simulink model "Grid_SensorLayout_SpatialAllignment_Clustering"  (R2018a)
settings: Solver=FixedStepAuto  StartTime=0.0  StopTime=SimulationTime  FixedStep=SamplingTime  RelTol=1e-3
values from neighbouring files (symbols this model uses):
  ValidateGRID = true    [SensorFusion_Script0_main.m]
  ValidateLAYOUT = true    [SensorFusion_Script0_main.m]
  VisualizeCLUSTERING = true    [SensorFusion_Script0_main.m]
undefined symbols (not defined in the file or in its folder): ACTIVATE_CAM, ACTIVATE_RAD, CAM1_detTimeStamp, CAM1_MeasNoise, CAM1_objClassID, CAM1_PX, CAM1_PY, CAM1_VX, CAM1_VY, CAM2_detTimeStamp, CAM2_MeasNoise, CAM2_objClassID, CAM2_PX, CAM2_PY, CAM2_VX, CAM2_VY, CAM3_detTimeStamp, CAM3_MeasNoise, CAM3_objClassID, CAM3_PX, CAM3_PY, CAM3_VX, CAM3_VY, CAM4_detTimeStamp, CAM4_MeasNoise, CAM4_objClassID, CAM4_PX, CAM4_PY, CAM4_VX, CAM4_VY, CAM5_detTimeStamp, CAM5_MeasNoise, CAM5_objClassID, CAM5_PX, CAM5_PY, CAM5_VX, CAM5_VY, CAM6_detTimeStamp, CAM6_MeasNoise, CAM6_objClassID, CAM6_PX, CAM6_PY, CAM6_VX, CAM6_VY, CAM7_detTimeStamp, CAM7_MeasNoise, CAM7_objClassID, CAM7_PX, CAM7_PY, CAM7_VX, CAM7_VY, CAM8_detTimeStamp, CAM8_MeasNoise, CAM8_objClassID, CAM8_PX, CAM8_PY, CAM8_VX, CAM8_VY, CAM_nMeas, CAM_TYPE ... (+171)
libraries: simulink_extras x4
(part 3 of 10)

== system Grid_SensorLayout_SpatialAllignment_Clustering/SENSOR_MEASUREMENTS/RADAR_CAMERA_EGO_SENSOR_INTERFACE/RoadSensors/LineSensor2 ==
  timeIdx : Inport
  nLines : Inport  Port=2
  CameraLineCoeff : Inport  Port=3
  ExtractMeasParam1 : Subsystem
  For Iterator : ForIterator  ResetStates=reset  IterationSource=external  IterationVariableDataType=int16
  IsValid2 : Subsystem
  Selector : Selector  InputPortWidth=nCameras  IndexOptions=Index vector (dialog)  Indices=2  OutputSizes=1
  Subsystem1 : Subsystem
  C1 : Outport
  wires:
  ExtractMeasParam1/7(xmax) -> Subsystem1/9(xmax)
  ExtractMeasParam1/8(lineMarkWidth) -> Subsystem1/10(lineWidth)
  [index] -> IsValid2/1(LineID), Subsystem1/12(iter), ExtractMeasParam1/1(idx)
  timeIdx/1 -> ExtractMeasParam1/2(time)
  ExtractMeasParam1/2(curvRate) -> IsValid2/3(curvatureRate), [curvRate]
  [curvRate] -> Subsystem1/3(curvRate)
  [curv] -> Subsystem1/2(curv)
  ExtractMeasParam1/3(curvLength) -> IsValid2/4(curvLength), [curvLen]
  ExtractMeasParam1/1(curvature) -> IsValid2/2(curvature), [curv]
  Subsystem1/1(C1) -> C1/1
  [curvLen] -> Subsystem1/4(curvLen)
  For Iterator/1 -> [index]
  ExtractMeasParam1/4(headingAngle) -> IsValid2/5(HeadingAngle), [alpha]
  ExtractMeasParam1/5(lateralOffset) -> Subsystem1/7(lateralOffset)
  Selector/1 -> For Iterator/1
  IsValid2/1(validID) -> Subsystem1/6(ValidID)
  ExtractMeasParam1/6(xmin) -> Subsystem1/8(xmin)
  CameraLineCoeff/1 -> Subsystem1/1(CameraLineCoeff)
  nLines/1 -> Selector/1
  ExtractMeasParam1/9(measCaptureTime) -> Subsystem1/11(TIME_STAMP)
  [alpha] -> Subsystem1/5(alpha)

== system Grid_SensorLayout_SpatialAllignment_Clustering/SENSOR_MEASUREMENTS/RADAR_CAMERA_EGO_SENSOR_INTERFACE/RoadSensors/LineSensor3 ==
  timeIdx : Inport
  nLines : Inport  Port=2
  CameraLineCoeff : Inport  Port=3
  ExtractMeasParam1 : Subsystem
  For Iterator : ForIterator  ResetStates=reset  IterationSource=external  IterationVariableDataType=int16
  IsValid2 : Subsystem
  Selector : Selector  InputPortWidth=nCameras  IndexOptions=Index vector (dialog)  Indices=3  OutputSizes=1
  Subsystem1 : Subsystem
  C1 : Outport
  wires:
  ExtractMeasParam1/7(xmax) -> Subsystem1/9(xmax)
  ExtractMeasParam1/8(lineMarkWidth) -> Subsystem1/10(lineWidth)
  [index] -> IsValid2/1(LineID), Subsystem1/12(iter), ExtractMeasParam1/1(idx)
  timeIdx/1 -> ExtractMeasParam1/2(time)
  ExtractMeasParam1/2(curvRate) -> IsValid2/3(curvatureRate), [curvRate]
  [curvRate] -> Subsystem1/3(curvRate)
  [curv] -> Subsystem1/2(curv)
  ExtractMeasParam1/3(curvLength) -> IsValid2/4(curvLength), [curvLen]
  ExtractMeasParam1/1(curvature) -> IsValid2/2(curvature), [curv]
  Subsystem1/1(C1) -> C1/1
  [curvLen] -> Subsystem1/4(curvLen)
  For Iterator/1 -> [index]
  ExtractMeasParam1/4(headingAngle) -> IsValid2/5(HeadingAngle), [alpha]
  ExtractMeasParam1/5(lateralOffset) -> Subsystem1/7(lateralOffset)
  Selector/1 -> For Iterator/1
  IsValid2/1(validID) -> Subsystem1/6(ValidID)
  ExtractMeasParam1/6(xmin) -> Subsystem1/8(xmin)
  CameraLineCoeff/1 -> Subsystem1/1(CameraLineCoeff)
  nLines/1 -> Selector/1
  ExtractMeasParam1/9(measCaptureTime) -> Subsystem1/11(TIME_STAMP)
  [alpha] -> Subsystem1/5(alpha)

== system Grid_SensorLayout_SpatialAllignment_Clustering/SENSOR_MEASUREMENTS/RADAR_CAMERA_EGO_SENSOR_INTERFACE/RoadSensors/LineSensor4 ==
  timeIdx : Inport
  nLines : Inport  Port=2
  CameraLineCoeff : Inport  Port=3
  ExtractMeasParam1 : Subsystem
  For Iterator : ForIterator  ResetStates=reset  IterationSource=external  IterationVariableDataType=int16
  IsValid2 : Subsystem
  Selector : Selector  InputPortWidth=nCameras  IndexOptions=Index vector (dialog)  Indices=4  OutputSizes=1
  Subsystem1 : Subsystem
  C1 : Outport
  wires:
  ExtractMeasParam1/7(xmax) -> Subsystem1/9(xmax)
  ExtractMeasParam1/8(lineMarkWidth) -> Subsystem1/10(lineWidth)
  [index] -> IsValid2/1(LineID), Subsystem1/12(iter), ExtractMeasParam1/1(idx)
  timeIdx/1 -> ExtractMeasParam1/2(time)
  ExtractMeasParam1/2(curvRate) -> IsValid2/3(curvatureRate), [curvRate]
  [curvRate] -> Subsystem1/3(curvRate)
  [curv] -> Subsystem1/2(curv)
  ExtractMeasParam1/3(curvLength) -> IsValid2/4(curvLength), [curvLen]
  ExtractMeasParam1/1(curvature) -> IsValid2/2(curvature), [curv]
  Subsystem1/1(C1) -> C1/1
  [curvLen] -> Subsystem1/4(curvLen)
  For Iterator/1 -> [index]
  ExtractMeasParam1/4(headingAngle) -> IsValid2/5(HeadingAngle), [alpha]
  ExtractMeasParam1/5(lateralOffset) -> Subsystem1/7(lateralOffset)
  Selector/1 -> For Iterator/1
  IsValid2/1(validID) -> Subsystem1/6(ValidID)
  ExtractMeasParam1/6(xmin) -> Subsystem1/8(xmin)
  CameraLineCoeff/1 -> Subsystem1/1(CameraLineCoeff)
  nLines/1 -> Selector/1
  ExtractMeasParam1/9(measCaptureTime) -> Subsystem1/11(TIME_STAMP)
  [alpha] -> Subsystem1/5(alpha)

== system Grid_SensorLayout_SpatialAllignment_Clustering/SENSOR_MEASUREMENTS/RADAR_CAMERA_EGO_SENSOR_INTERFACE/RoadSensors/LineSensor5 ==
  timeIdx : Inport
  nLines : Inport  Port=2
  CameraLineCoeff : Inport  Port=3
  ExtractMeasParam1 : Subsystem
  For Iterator : ForIterator  ResetStates=reset  IterationSource=external  IterationVariableDataType=int16
  IsValid2 : Subsystem
  Selector : Selector  InputPortWidth=nCameras  IndexOptions=Index vector (dialog)  Indices=5  OutputSizes=1
  Subsystem1 : Subsystem
  C1 : Outport
  wires:
  ExtractMeasParam1/7(xmax) -> Subsystem1/9(xmax)
  ExtractMeasParam1/8(lineMarkWidth) -> Subsystem1/10(lineWidth)
  [index] -> IsValid2/1(LineID), Subsystem1/12(iter), ExtractMeasParam1/1(idx)
  timeIdx/1 -> ExtractMeasParam1/2(time)
  ExtractMeasParam1/2(curvRate) -> IsValid2/3(curvatureRate), [curvRate]
  [curvRate] -> Subsystem1/3(curvRate)
  [curv] -> Subsystem1/2(curv)
  ExtractMeasParam1/3(curvLength) -> IsValid2/4(curvLength), [curvLen]
  ExtractMeasParam1/1(curvature) -> IsValid2/2(curvature), [curv]
  Subsystem1/1(C1) -> C1/1
  [curvLen] -> Subsystem1/4(curvLen)
  For Iterator/1 -> [index]
  ExtractMeasParam1/4(headingAngle) -> IsValid2/5(HeadingAngle), [alpha]
  ExtractMeasParam1/5(lateralOffset) -> Subsystem1/7(lateralOffset)
  Selector/1 -> For Iterator/1
  IsValid2/1(validID) -> Subsystem1/6(ValidID)
  ExtractMeasParam1/6(xmin) -> Subsystem1/8(xmin)
  CameraLineCoeff/1 -> Subsystem1/1(CameraLineCoeff)
  nLines/1 -> Selector/1
  ExtractMeasParam1/9(measCaptureTime) -> Subsystem1/11(TIME_STAMP)
  [alpha] -> Subsystem1/5(alpha)

== system Grid_SensorLayout_SpatialAllignment_Clustering/SENSOR_MEASUREMENTS/RADAR_CAMERA_EGO_SENSOR_INTERFACE/RoadSensors/LineSensor6 ==
  timeIdx : Inport
  nLines : Inport  Port=2
  CameraLineCoeff : Inport  Port=3
  ExtractMeasParam1 : Subsystem
  For Iterator : ForIterator  ResetStates=reset  IterationSource=external  IterationVariableDataType=int16
  IsValid2 : Subsystem
  Selector : Selector  InputPortWidth=nCameras  IndexOptions=Index vector (dialog)  Indices=6  OutputSizes=1
  Subsystem1 : Subsystem
  C1 : Outport
  wires:
  ExtractMeasParam1/7(xmax) -> Subsystem1/9(xmax)
  ExtractMeasParam1/8(lineMarkWidth) -> Subsystem1/10(lineWidth)
  [index] -> IsValid2/1(LineID), Subsystem1/12(iter), ExtractMeasParam1/1(idx)
  timeIdx/1 -> ExtractMeasParam1/2(time)
  ExtractMeasParam1/2(curvRate) -> IsValid2/3(curvatureRate), [curvRate]
  [curvRate] -> Subsystem1/3(curvRate)
  [curv] -> Subsystem1/2(curv)
  ExtractMeasParam1/3(curvLength) -> IsValid2/4(curvLength), [curvLen]
  ExtractMeasParam1/1(curvature) -> IsValid2/2(curvature), [curv]
  Subsystem1/1(C1) -> C1/1
  [curvLen] -> Subsystem1/4(curvLen)
  For Iterator/1 -> [index]
  ExtractMeasParam1/4(headingAngle) -> IsValid2/5(HeadingAngle), [alpha]
  ExtractMeasParam1/5(lateralOffset) -> Subsystem1/7(lateralOffset)
  Selector/1 -> For Iterator/1
  IsValid2/1(validID) -> Subsystem1/6(ValidID)
  ExtractMeasParam1/6(xmin) -> Subsystem1/8(xmin)
  CameraLineCoeff/1 -> Subsystem1/1(CameraLineCoeff)
  nLines/1 -> Selector/1
  ExtractMeasParam1/9(measCaptureTime) -> Subsystem1/11(TIME_STAMP)
  [alpha] -> Subsystem1/5(alpha)

== system Grid_SensorLayout_SpatialAllignment_Clustering/SENSOR_MEASUREMENTS/RADAR_CAMERA_EGO_SENSOR_INTERFACE/RoadSensors/LineSensor7 ==
  timeIdx : Inport
  nLines : Inport  Port=2
  CameraLineCoeff : Inport  Port=3
  ExtractMeasParam1 : Subsystem
  For Iterator : ForIterator  ResetStates=reset  IterationSource=external  IterationVariableDataType=int16
  IsValid2 : Subsystem
  Selector : Selector  InputPortWidth=nCameras  IndexOptions=Index vector (dialog)  Indices=7  OutputSizes=1
  Subsystem1 : Subsystem
  C1 : Outport
  wires:
  ExtractMeasParam1/7(xmax) -> Subsystem1/9(xmax)
  ExtractMeasParam1/8(lineMarkWidth) -> Subsystem1/10(lineWidth)
  [index] -> IsValid2/1(LineID), Subsystem1/12(iter), ExtractMeasParam1/1(idx)
  timeIdx/1 -> ExtractMeasParam1/2(time)
  ExtractMeasParam1/2(curvRate) -> IsValid2/3(curvatureRate), [curvRate]
  [curvRate] -> Subsystem1/3(curvRate)
  [curv] -> Subsystem1/2(curv)
  ExtractMeasParam1/3(curvLength) -> IsValid2/4(curvLength), [curvLen]
  ExtractMeasParam1/1(curvature) -> IsValid2/2(curvature), [curv]
  Subsystem1/1(C1) -> C1/1
  [curvLen] -> Subsystem1/4(curvLen)
  For Iterator/1 -> [index]
  ExtractMeasParam1/4(headingAngle) -> IsValid2/5(HeadingAngle), [alpha]
  ExtractMeasParam1/5(lateralOffset) -> Subsystem1/7(lateralOffset)
  Selector/1 -> For Iterator/1
  IsValid2/1(validID) -> Subsystem1/6(ValidID)
  ExtractMeasParam1/6(xmin) -> Subsystem1/8(xmin)
  CameraLineCoeff/1 -> Subsystem1/1(CameraLineCoeff)
  nLines/1 -> Selector/1
  ExtractMeasParam1/9(measCaptureTime) -> Subsystem1/11(TIME_STAMP)
  [alpha] -> Subsystem1/5(alpha)

== system Grid_SensorLayout_SpatialAllignment_Clustering/SENSOR_MEASUREMENTS/RADAR_CAMERA_EGO_SENSOR_INTERFACE/RoadSensors/LineSensor8 ==
  timeIdx : Inport
  nLines : Inport  Port=2
  CameraLineCoeff : Inport  Port=3
  ExtractMeasParam1 : Subsystem
  For Iterator : ForIterator  ResetStates=reset  IterationSource=external  IterationVariableDataType=int16
  IsValid2 : Subsystem
  Selector : Selector  InputPortWidth=nCameras  IndexOptions=Index vector (dialog)  Indices=8  OutputSizes=1
  Subsystem1 : Subsystem
  C1 : Outport
  wires:
  ExtractMeasParam1/7(xmax) -> Subsystem1/9(xmax)
  ExtractMeasParam1/8(lineMarkWidth) -> Subsystem1/10(lineWidth)
  [index] -> IsValid2/1(LineID), Subsystem1/12(iter), ExtractMeasParam1/1(idx)
  timeIdx/1 -> ExtractMeasParam1/2(time)
  ExtractMeasParam1/2(curvRate) -> IsValid2/3(curvatureRate), [curvRate]
  [curvRate] -> Subsystem1/3(curvRate)
  [curv] -> Subsystem1/2(curv)
  ExtractMeasParam1/3(curvLength) -> IsValid2/4(curvLength), [curvLen]
  ExtractMeasParam1/1(curvature) -> IsValid2/2(curvature), [curv]
  Subsystem1/1(C1) -> C1/1
  [curvLen] -> Subsystem1/4(curvLen)
  For Iterator/1 -> [index]
  ExtractMeasParam1/4(headingAngle) -> IsValid2/5(HeadingAngle), [alpha]
  ExtractMeasParam1/5(lateralOffset) -> Subsystem1/7(lateralOffset)
  Selector/1 -> For Iterator/1
  IsValid2/1(validID) -> Subsystem1/6(ValidID)
  ExtractMeasParam1/6(xmin) -> Subsystem1/8(xmin)
  CameraLineCoeff/1 -> Subsystem1/1(CameraLineCoeff)
  nLines/1 -> Selector/1
  ExtractMeasParam1/9(measCaptureTime) -> Subsystem1/11(TIME_STAMP)
  [alpha] -> Subsystem1/5(alpha)

== system Grid_SensorLayout_SpatialAllignment_Clustering/OBJECT_TRACKER_SENSOR_FUSION/NEAREST_NEIGHBOUR_FOR_CAMERA_MEASUREMENT_GROUPING/NN_MEASUREMENT_GROUPING_WITHIN_EPS/COMPUTE_MEAN_IF_CLUSTER_FORMED/COMPUTE_COVARIANCE1 ==
  covariance_sum : Inport
  n : Inport  Port=2
  Constant : Constant  Value=uint16(1)
  Constant1 : Constant  Value=uint16(0)
  Constant2 : Constant  Value=single(eye(2))
  Constant3 : Constant  Value=single(0.001)
  Divide : Product  Inputs=*/
  LessThanOrEqual : RelationalOperator  Operator=>  OutDataTypeStr=boolean  RndMeth=Simplest
  LessThanOrEqual1 : RelationalOperator  Operator=<=  OutDataTypeStr=boolean  RndMeth=Simplest
  Logical Operator : Logic  AllPortsSameDT=off  OutDataTypeStr=boolean
  Selector : Selector  NumberOfDimensions=2  InputPortWidth=3  IndexOptions=Index vector (dialog),Index vector (dialog)  Indices=1,1  OutputSizes=1,1
  Selector1 : Selector  NumberOfDimensions=2  InputPortWidth=3  IndexOptions=Index vector (dialog),Index vector (dialog)  Indices=1,1  OutputSizes=1,1
  Subtract : Sum  Inputs=-+
  Switch : Switch  Criteria=u2 > Threshold  Threshold=uint16(1)
  Switch1 : Switch  Criteria=u2 > Threshold  Threshold=uint16(1)
  Covariance : Outport
  wires:
  n/1 -> [nPts], Switch/2
  Constant/1 -> Switch/1
  covariance_sum/1 -> Divide/1
  Constant1/1 -> Switch/3
  Switch/1 -> Subtract/1
  [nPts] -> Subtract/2
  Subtract/1 -> Divide/2
  Logical Operator/1 -> Switch1/2
  Switch1/1 -> Covariance/1
  Constant2/1 -> Switch1/3
  Divide/1 -> Selector1/1, Switch1/1, Selector/1
  Selector/1 -> LessThanOrEqual/1
  Selector1/1 -> LessThanOrEqual1/2
  Constant3/1 -> LessThanOrEqual1/1, LessThanOrEqual/2
  LessThanOrEqual/1 -> Logical Operator/1
  LessThanOrEqual1/1 -> Logical Operator/2

== system Grid_SensorLayout_SpatialAllignment_Clustering/OBJECT_TRACKER_SENSOR_FUSION/NEAREST_NEIGHBOUR_FOR_CAMERA_MEASUREMENT_GROUPING/NN_MEASUREMENT_GROUPING_WITHIN_EPS/COMPUTE_MEAN_IF_CLUSTER_FORMED/COMPUTE_COVARIANCE_SUM ==
  mean : Inport
  MeasArray : Inport  Port=2
  nPoints : Inport  Port=3
  ClusterMembers : Inport  Port=4
  Add1 : Sum
  Bus Selector : BusSelector  OutputSignals=MeasArray
  For Iterator : ForIterator  ResetStates=reset  IterationSource=external
  Matrix Multiply : Product  Multiplication=Matrix(*)
  Selector : Selector  NumberOfDimensions=2  InputPortWidth=3  IndexOptions=Select all,Index vector (port)  Indices=[1 3],1  OutputSizes=1,1
  Selector1 : Selector  NumberOfDimensions=2  InputPortWidth=3  IndexOptions=Select all,Index vector (port)  Indices=[1 3],1  OutputSizes=1,1
  Subtract : Sum  Inputs=+-
  Transpose : Math  Operator=transpose  SaturateOnIntegerOverflow=on
  Unit Delay : UnitDelay  InitialCondition=single(zeros(2,2))  SampleTime=-1
  ClusterCovSUM : Outport
  wires:
  nPoints/1 -> For Iterator/1
  ClusterMembers/1 -> Selector/1
  For Iterator/1 -> Selector/2
  MeasArray/1 -> Bus Selector/1
  Bus Selector/1 -> Selector1/1  "<MeasArray>"
  Selector/1 -> Selector1/2
  Unit Delay/1 -> Add1/1
  Add1/1 -> Unit Delay/1, ClusterCovSUM/1
  Subtract/1 -> Matrix Multiply/1, Transpose/1
  Transpose/1 -> Matrix Multiply/2
  Matrix Multiply/1 -> Add1/2
  Selector1/1 -> Subtract/2
  mean/1 -> Subtract/1

== system Grid_SensorLayout_SpatialAllignment_Clustering/OBJECT_TRACKER_SENSOR_FUSION/NEAREST_NEIGHBOUR_FOR_CAMERA_MEASUREMENT_GROUPING/NN_MEASUREMENT_GROUPING_WITHIN_EPS/COMPUTE_MEAN_IF_CLUSTER_FORMED/COMPUTE_MEAN ==
  mean_sum : Inport
  n : Inport  Port=2
  Divide : Product  Inputs=*/
  mean : Outport
  wires:
  mean_sum/1 -> Divide/1
  Divide/1 -> mean/1
  n/1 -> Divide/2

== system Grid_SensorLayout_SpatialAllignment_Clustering/OBJECT_TRACKER_SENSOR_FUSION/NEAREST_NEIGHBOUR_FOR_CAMERA_MEASUREMENT_GROUPING/NN_MEASUREMENT_GROUPING_WITHIN_EPS/COMPUTE_MEAN_IF_CLUSTER_FORMED/COMPUTE_MEAN_SUM ==
  ClusterMembers : Inport
  nPoints : Inport  Port=2
  MeasArray : Inport  Port=3
  Add1 : Sum
  Bus Selector : BusSelector  OutputSignals=MeasArray
  For Iterator : ForIterator  ResetStates=reset  IterationSource=external
  Selector : Selector  NumberOfDimensions=2  InputPortWidth=3  IndexOptions=Select all,Index vector (port)  Indices=[1 3],1  OutputSizes=1,1
  Selector1 : Selector  NumberOfDimensions=2  InputPortWidth=3  IndexOptions=Select all,Index vector (port)  Indices=[1 3],1  OutputSizes=1,1
  Unit Delay : UnitDelay  InitialCondition=single(0)  SampleTime=-1
  ClusterMeanSUM : Outport
  wires:
  nPoints/1 -> For Iterator/1
  ClusterMembers/1 -> Selector/1
  For Iterator/1 -> Selector/2
  MeasArray/1 -> Bus Selector/1
  Bus Selector/1 -> Selector1/1  "<MeasArray>"
  Selector/1 -> Selector1/2
  Selector1/1 -> Add1/2
  Unit Delay/1 -> Add1/1
  Add1/1 -> ClusterMeanSUM/1, Unit Delay/1

== system Grid_SensorLayout_SpatialAllignment_Clustering/OBJECT_TRACKER_SENSOR_FUSION/NEAREST_NEIGHBOUR_FOR_CAMERA_MEASUREMENT_GROUPING/NN_MEASUREMENT_GROUPING_WITHIN_EPS/COMPUTE_MEAN_IF_CLUSTER_FORMED/GET_DATA ==
  CLSTR : Inport
  Bus Selector : BusSelector  OutputSignals=ClusterSizes,nClusters,ClusterMember
  Selector : Selector  NumberOfDimensions=2  InputPortWidth=3  IndexOptions=Select all,Index vector (port)  Indices=[1 3],1  OutputSizes=1,1
  nPts : Outport
  <ClusterMember> : Outport  Port=2
  wires:
  Bus Selector/1 -> Selector/1  "<ClusterSizes>"
  Selector/1 -> nPts/1
  Bus Selector/2 -> Selector/2  "<nClusters>"
  Bus Selector/3 -> <ClusterMember>/1  "<ClusterMember>"
  CLSTR/1 -> Bus Selector/1

== system Grid_SensorLayout_SpatialAllignment_Clustering/OBJECT_TRACKER_SENSOR_FUSION/NEAREST_NEIGHBOUR_FOR_CAMERA_MEASUREMENT_GROUPING/NN_MEASUREMENT_GROUPING_WITHIN_EPS/For Iterator Subsystem/If Action Subsystem ==
  CLSTR_DATA : Inport
  Action Port : ActionPort  ActionType=else
  Constant : Constant  Value=uint16(0)
  CLSTR_DATA_NO_UPD : Outport
  nPtsEpsNoUpd : Outport  Port=2
  wires:
  CLSTR_DATA/1 -> CLSTR_DATA_NO_UPD/1
  Constant/1 -> nPtsEpsNoUpd/1

== system Grid_SensorLayout_SpatialAllignment_Clustering/OBJECT_TRACKER_SENSOR_FUSION/NEAREST_NEIGHBOUR_FOR_CAMERA_MEASUREMENT_GROUPING/NN_MEASUREMENT_GROUPING_WITHIN_EPS/For Iterator Subsystem/MERGE_SIGNALS ==
  CLSTR_NO_UPD : Inport
  nPtsEpsNoUpd : Inport  Port=2
  nPtsUpd : Inport  Port=3
  CLSTR_UPD : Inport  Port=4
  Merge : Merge
  Merge1 : Merge
  nPtsEps : Outport
  CLSTR_DATA : Outport  Port=2
  wires:
  CLSTR_NO_UPD/1 -> Merge1/1
  Merge1/1 -> CLSTR_DATA/1
  nPtsEpsNoUpd/1 -> Merge/1
  Merge/1 -> nPtsEps/1
  nPtsUpd/1 -> Merge/2
  CLSTR_UPD/1 -> Merge1/2

== system Grid_SensorLayout_SpatialAllignment_Clustering/OBJECT_TRACKER_SENSOR_FUSION/NEAREST_NEIGHBOUR_FOR_CAMERA_MEASUREMENT_GROUPING/NN_MEASUREMENT_GROUPING_WITHIN_EPS/For Iterator Subsystem/NN ==
  CLSTR_DATA : Inport  OutDataTypeStr=Bus: CLUSTER_DATA_STRUCT_SNSR
  measArray : Inport  Port=2
  idx_i : Inport  Port=3
  Action Port : ActionPort  ActionType=then
  PERFORM_NN_CLUSTERING : Subsystem
  SET_CLUSTER_ID_AND_UPDATE_NUMBER_OF_CLUSTERS : Subsystem
  Subsystem : Subsystem
  nPtsEps : Outport
  CLSTR_DATA_UPD : Outport  Port=2
  wires:
  idx_i/1 -> PERFORM_NN_CLUSTERING/4(idx_i)
  SET_CLUSTER_ID_AND_UPDATE_NUMBER_OF_CLUSTERS/2(CLUSTER_DATA) -> PERFORM_NN_CLUSTERING/3(CLSTR_DATA)
  SET_CLUSTER_ID_AND_UPDATE_NUMBER_OF_CLUSTERS/1(nRadMeas) -> PERFORM_NN_CLUSTERING/1(nMeas)
  CLSTR_DATA/1 -> SET_CLUSTER_ID_AND_UPDATE_NUMBER_OF_CLUSTERS/1(CLUSTERING_DATA)
  measArray/1 -> SET_CLUSTER_ID_AND_UPDATE_NUMBER_OF_CLUSTERS/2(CAM_MEAS_CTS), [meas]
  [meas] -> PERFORM_NN_CLUSTERING/2(measArray)
  Subsystem/1(ClstrSize) -> nPtsEps/1
  PERFORM_NN_CLUSTERING/1(CLSTR_DATA_UPD) -> Subsystem/1(CLSTR_DATA), CLSTR_DATA_UPD/1

== system Grid_SensorLayout_SpatialAllignment_Clustering/OBJECT_TRACKER_SENSOR_FUSION/NEAREST_NEIGHBOUR_FOR_CAMERA_MEASUREMENT_GROUPING/NN_MEASUREMENT_GROUPING_WITHIN_EPS/For Iterator Subsystem/Subsystem ==
  idx_i : Inport
  CLSTR_in : Inport  Port=2
  Bus Selector : BusSelector  OutputSignals=isMeasVisitedFlag
  Logical Operator1 : Logic  Operator=NOT  AllPortsSameDT=off  OutDataTypeStr=boolean
  Selector1 : Selector  NumberOfDimensions=2  InputPortWidth=3  IndexOptions=Select all,Index vector (port)  Indices=1,1  OutputSizes=1,1
  Unit Delay : UnitDelay  InitialCondition=CLSTR_SNSR_DELAY_INIT  SampleTime=-1
  isNotVisited : Outport
  CLSTR_out : Outport  Port=2
  wires:
  Logical Operator1/1 -> isNotVisited/1
  Selector1/1 -> Logical Operator1/1
  idx_i/1 -> Selector1/2
  CLSTR_in/1 -> Unit Delay/1
  Bus Selector/1 -> Selector1/1  "<isMeasVisitedFlag>"
  Unit Delay/1 -> CLSTR_out/1, Bus Selector/1

== system Grid_SensorLayout_SpatialAllignment_Clustering/OBJECT_TRACKER_SENSOR_FUSION/NEAREST_NEIGHBOUR_FOR_CAMERA_MEASUREMENT_GROUPING/NN_MEASUREMENT_GROUPING_WITHIN_EPS/Subsystem3/GET_DATA_FROM_BUS ==
  CLSTR_DATA : Inport
  Bus Selector : BusSelector  OutputSignals=ClusterCenter,ClusterCovariance,nClusters
  <ClusterCenter> : Outport
  <ClusterCovariance> : Outport  Port=2
  <nClusters> : Outport  Port=3
  wires:
  Bus Selector/3 -> <nClusters>/1  "<nClusters>"
  Bus Selector/1 -> <ClusterCenter>/1  "<ClusterCenter>"
  CLSTR_DATA/1 -> Bus Selector/1
  Bus Selector/2 -> <ClusterCovariance>/1  "<ClusterCovariance>"

== system Grid_SensorLayout_SpatialAllignment_Clustering/OBJECT_TRACKER_SENSOR_FUSION/NEAREST_NEIGHBOUR_FOR_CAMERA_MEASUREMENT_GROUPING/NN_MEASUREMENT_GROUPING_WITHIN_EPS/Subsystem3/SET_DATA_TO_BUS ==
  CLSTR_DATA : Inport
  Mean_ARRAY : Inport  Port=2
  Cov_ARRAY : Inport  Port=3
  Bus Creator : BusCreator  Inputs=7  OutDataTypeStr=Bus: CLUSTER_DATA_STRUCT_SNSR  NonVirtualBus=on
      settings: InheritFromInputs=off
  Bus Selector1 : BusSelector  OutputSignals=ClusterCenter,ClusterCovariance,ClusterSizes,ClusterToMeasAssignment,isMeasVisitedFlag,nClusters,ClusterMember
  Constant1 : Constant  Value=ClusterMemArray_SNSR
  Reshape1 : Reshape  OutputDimensionality=Row vector (2-D)
  Terminator1 : Terminator
  Terminator2 : Terminator
  Terminator3 : Terminator
  "CLSTR_DATA_UPD " : Outport
  wires:
  Constant1/1 -> Reshape1/1  "ClusterMember"
  Bus Selector1/5 -> Bus Creator/5  "<isMeasVisitedFlag>"
  Cov_ARRAY/1 -> Bus Creator/2  "ClusterCovariance"
  Mean_ARRAY/1 -> Bus Creator/1  "ClusterCenter"
  Bus Selector1/1 -> Terminator2/1  "<ClusterCenter>"
  Bus Selector1/7 -> Terminator1/1  "<ClusterMember>"
  Bus Selector1/2 -> Terminator3/1  "<ClusterCovariance>"
  Bus Selector1/3 -> Bus Creator/3  "<ClusterSizes>"
  Reshape1/1 -> Bus Creator/7  "ClusterMember"
  Bus Selector1/4 -> Bus Creator/4  "<ClusterToMeasAssignment>"
  Bus Selector1/6 -> Bus Creator/6  "<nClusters>"
  Bus Creator/1 -> "CLSTR_DATA_UPD "/1
  CLSTR_DATA/1 -> Bus Selector1/1

== system Grid_SensorLayout_SpatialAllignment_Clustering/OBJECT_TRACKER_SENSOR_FUSION/NEAREST_NEIGHBOUR_FOR_CAMERA_MEASUREMENT_GROUPING/NN_MEASUREMENT_GROUPING_WITHIN_EPS/Subsystem3/UPDATE_CLUSTER_DATA ==
  Center_ARRAY : Inport
  Cov_ARRAY : Inport  Port=2
  ID : Inport  Port=3
  mean1 : Inport  Port=4
  mean2 : Inport  Port=5
  Cov1 : Inport  Port=6
  Cov2 : Inport  Port=7
  FLAG : Inport  Port=8
  Assignment : Assignment  NumberOfDimensions=2  DiagnosticForDimensions=Warning  IndexOptions=Assign all,Index vector (port)  Indices=1,1  OutputSizes=1,1
  Assignment1 : Assignment  NumberOfDimensions=3  DiagnosticForDimensions=Warning  IndexOptions=Assign all,Assign all,Index vector (port)  Indices=1,1,1  OutputSizes=1,1,1
  Merge : Merge
  Merge2 : Merge
  Selector : Selector  NumberOfDimensions=2  InputPortWidth=3  IndexOptions=Select all,Index vector (port)  Indices=[1 3],1  OutputSizes=1,1
  Selector1 : Selector  NumberOfDimensions=3  InputPortWidth=3  IndexOptions=Select all,Select all,Index vector (port)  Indices=[1 3],1,1  OutputSizes=1,1,1
  Switch : Switch  Criteria=u2 ~= 0
  Switch1 : Switch  Criteria=u2 ~= 0
  CenterUpd : Outport
  CovUpd : Outport  Port=2
  wires:
  Selector/1 -> Switch/3
  Merge2/1 -> Switch1/1
  Cov_ARRAY/1 -> Assignment1/1, Selector1/1
  mean1/1 -> Merge/1
  Selector1/1 -> Switch1/3
  Merge/1 -> Switch/1
  Switch1/1 -> Assignment1/2
  Switch/1 -> Assignment/2
  Cov2/1 -> Merge2/2
  Assignment1/1 -> CovUpd/1
  Assignment/1 -> CenterUpd/1
  Cov1/1 -> Merge2/1
  mean2/1 -> Merge/2
  FLAG/1 -> [FLAG]
  [FLAG] -> Switch/2
  [FLAG] -> Switch1/2
  [ID] -> Assignment/3, Selector/2
  ID/1 -> [ID], Assignment1/3, Selector1/2
  Center_ARRAY/1 -> Selector/1, Assignment/1

== system Grid_SensorLayout_SpatialAllignment_Clustering/OBJECT_TRACKER_SENSOR_FUSION/SENSOR_LAYOUT_AND_CHRACTERIZATION/PRE_COMPUTE_SENSOR_FOV_GRID/COMPUTE_CAMERA_SNSR_GRID/ComputeCoverageANDConfidence ==
  RegionConfidenceArray : Inport
  nGridCells : Inport  Port=2
  GridIDVector : Inport  Port=3
  GridParam : Inport  Port=4
  SensorID : Inport  Port=5
  SensorExtrinsic : Inport  Port=6
  SensorIntrinsic : Inport  Port=7
  FOVOverlapArray : Inport  Port=8
  Compute_Cell_X_and_Y_index : Subsystem
  For Iterator : ForIterator  ResetStates=reset  IterationSource=external
  SET_DATA : Subsystem
  RegionConfidence : Outport
  FOVOverlap : Outport  Port=2
  wires:
  nGridCells/1 -> For Iterator/1
  For Iterator/1 -> SET_DATA/1(GridIndex), Compute_Cell_X_and_Y_index/1(CellIndex)
  GridParam/1 -> Compute_Cell_X_and_Y_index/3(GridParam)
  GridIDVector/1 -> Compute_Cell_X_and_Y_index/2(GridID_vec)
  SensorExtrinsic/1 -> Compute_Cell_X_and_Y_index/4(SensorExtrinsicParam)
  SensorIntrinsic/1 -> Compute_Cell_X_and_Y_index/5(SensorIntrinsicParam)
  RegionConfidenceArray/1 -> SET_DATA/2(RegionConfiArray)
  Compute_Cell_X_and_Y_index/1(RegionConfidence) -> SET_DATA/5(confi)
  SensorID/1 -> SET_DATA/4(SnsrIndex)
  FOVOverlapArray/1 -> SET_DATA/3(FOVOverlapArray)
  Compute_Cell_X_and_Y_index/2(FOVOverlap) -> SET_DATA/6(overlap)
  SET_DATA/1(RegionConfidence) -> RegionConfidence/1
  SET_DATA/2(FOVOverlap) -> FOVOverlap/1

== system Grid_SensorLayout_SpatialAllignment_Clustering/OBJECT_TRACKER_SENSOR_FUSION/SENSOR_LAYOUT_AND_CHRACTERIZATION/PRE_COMPUTE_SENSOR_FOV_GRID/COMPUTE_CAMERA_SNSR_GRID/GET_SENSOR_PARAMETERS ==
  SensorID : Inport
  SensorParam : Inport  Port=2
  Bus Selector : BusSelector  OutputSignals=CameraIntrinsics,CameraExtrinsics
  Bus Selector1 : BusSelector  OutputSignals=CameraType
  Selector : Selector  NumberOfDimensions=2  InputPortWidth=3  IndexOptions=Select all,Index vector (port)  Indices=[1 3],1  OutputSizes=1,1
  Selector1 : Selector  NumberOfDimensions=2  InputPortWidth=3  IndexOptions=Select all,Index vector (port)  Indices=[1 3],1  OutputSizes=1,1
  extrinsic : Outport
  intrinsic : Outport  Port=2
  wires:
  Bus Selector/2 -> Selector/1  "<CameraExtrinsics>"
  Bus Selector1/1 -> Selector1/2  "<CameraType>"
  Selector/1 -> extrinsic/1, Bus Selector1/1
  SensorID/1 -> Selector/2
  SensorParam/1 -> Bus Selector/1
  Bus Selector/1 -> Selector1/1  "<CameraIntrinsics>"
  Selector1/1 -> intrinsic/1

== system Grid_SensorLayout_SpatialAllignment_Clustering/OBJECT_TRACKER_SENSOR_FUSION/SENSOR_LAYOUT_AND_CHRACTERIZATION/PRE_COMPUTE_SENSOR_FOV_GRID/COMPUTE_RADAR_SNSR_GRID/ComputeCoverageANDConfidence ==
  RegionConfidenceArray : Inport
  nGridCells : Inport  Port=2
  GridIDVector : Inport  Port=3
  GridParam : Inport  Port=4
  SensorID : Inport  Port=5
  SensorExtrinsic : Inport  Port=6
  SensorIntrinsic : Inport  Port=7
  FOVOverlapArray : Inport  Port=8
  Compute_Cell_X_and_Y_index : Subsystem
  For Iterator : ForIterator  ResetStates=reset  IterationSource=external
  SET_DATA : Subsystem
  RegionConfidence : Outport
  FOVOverlap : Outport  Port=2
  wires:
  nGridCells/1 -> For Iterator/1
  For Iterator/1 -> SET_DATA/1(GridIndex), Compute_Cell_X_and_Y_index/1(CellIndex)
  GridParam/1 -> Compute_Cell_X_and_Y_index/3(GridParam)
  GridIDVector/1 -> Compute_Cell_X_and_Y_index/2(GridID_vec)
  SensorExtrinsic/1 -> Compute_Cell_X_and_Y_index/4(SensorExtrinsicParam)
  SensorIntrinsic/1 -> Compute_Cell_X_and_Y_index/5(SensorIntrinsicParam)
  RegionConfidenceArray/1 -> SET_DATA/2(RegionConfiArray)
  Compute_Cell_X_and_Y_index/1(RegionConfidence) -> SET_DATA/5(confi)
  SensorID/1 -> SET_DATA/4(SnsrIndex)
  FOVOverlapArray/1 -> SET_DATA/3(FOVOverlapArray)
  Compute_Cell_X_and_Y_index/2(FOVOverlap) -> SET_DATA/6(overlap)
  SET_DATA/1(RegionConfidence) -> RegionConfidence/1
  SET_DATA/2(FOVOverlap) -> FOVOverlap/1

== system Grid_SensorLayout_SpatialAllignment_Clustering/OBJECT_TRACKER_SENSOR_FUSION/SENSOR_LAYOUT_AND_CHRACTERIZATION/PRE_COMPUTE_SENSOR_FOV_GRID/COMPUTE_RADAR_SNSR_GRID/GET_SENSOR_PARAMETERS ==
  SensorID : Inport
  SensorParam : Inport  Port=2
  Bus Selector : BusSelector  OutputSignals=RadarIntrinsics,RadarExtrinsics
  Bus Selector1 : BusSelector  OutputSignals=RadarType
  Selector : Selector  NumberOfDimensions=2  InputPortWidth=3  IndexOptions=Select all,Index vector (port)  Indices=[1 3],1  OutputSizes=1,1
  Selector1 : Selector  NumberOfDimensions=2  InputPortWidth=3  IndexOptions=Select all,Index vector (port)  Indices=[1 3],1  OutputSizes=1,1
  extrinsic : Outport
  intrinsic : Outport  Port=2
  wires:
  Bus Selector/2 -> Selector/1  "<RadarExtrinsics>"
  Bus Selector1/1 -> Selector1/2  "<RadarType>"
  Selector/1 -> extrinsic/1, Bus Selector1/1
  SensorID/1 -> Selector/2
  SensorParam/1 -> Bus Selector/1
  Bus Selector/1 -> Selector1/1  "<RadarIntrinsics>"
  Selector1/1 -> intrinsic/1

== system Grid_SensorLayout_SpatialAllignment_Clustering/OBJECT_TRACKER_SENSOR_FUSION/SENSOR_LAYOUT_AND_CHRACTERIZATION/PRE_COMPUTE_SENSOR_FOV_GRID/CREATE_GRID/For Iterator Subsystem ==
  xIndex : Inport
  Cy : Inport  Port=2
  GridParam : Inport  Port=3
  CellIDArray : Inport  Port=4
  Compute_Grid_Cell_Cartesian_Coordinate : Subsystem
  Compute_Grid_Cell_Discreete_Index : Subsystem
  For Iterator : ForIterator  ResetStates=reset  IterationSource=external
  SET_DATA : Subsystem
  Terminator : Terminator
  Terminator1 : Terminator
  CellIDVectorUpd : Outport
  wires:
  Cy/1 -> For Iterator/1
  xIndex/1 -> Compute_Grid_Cell_Cartesian_Coordinate/2(x_Index)
  GridParam/1 -> Compute_Grid_Cell_Cartesian_Coordinate/1(GridParam), Compute_Grid_Cell_Discreete_Index/1(GridParam)
  Compute_Grid_Cell_Cartesian_Coordinate/2(y_Coordinate) -> Compute_Grid_Cell_Discreete_Index/3(y_coord)
  Compute_Grid_Cell_Cartesian_Coordinate/1(x_Coordinate) -> Compute_Grid_Cell_Discreete_Index/2(x_coord)
  For Iterator/1 -> Compute_Grid_Cell_Cartesian_Coordinate/3(y_Index)
  CellIDArray/1 -> SET_DATA/1(CellIDArray)
  SET_DATA/1(CellIDArrayUpd) -> CellIDVectorUpd/1
  Compute_Grid_Cell_Discreete_Index/1(CellID_x) -> Terminator/1
  Compute_Grid_Cell_Discreete_Index/2(CellID_y) -> Terminator1/1
  Compute_Grid_Cell_Discreete_Index/3(CellID) -> SET_DATA/2(CellID)

== system Grid_SensorLayout_SpatialAllignment_Clustering/OBJECT_TRACKER_SENSOR_FUSION/SENSOR_LAYOUT_AND_CHRACTERIZATION/SET_SENSOR_CALLIBRATION_PARAMETER/SET_CAMERA_SENSOR_PARAM/GET_DATA ==
  CAMSnsrParam : Inport
  Bus Selector : BusSelector  OutputSignals=CameraIntrinsics,CameraExtrinsics
  CameraIntrinsics : Outport
  CameraExtrinsics : Outport  Port=2
  wires:
  CAMSnsrParam/1 -> Bus Selector/1
  Bus Selector/2 -> CameraExtrinsics/1  "<CameraExtrinsics>"
  Bus Selector/1 -> CameraIntrinsics/1  "<CameraIntrinsics>"

== system Grid_SensorLayout_SpatialAllignment_Clustering/OBJECT_TRACKER_SENSOR_FUSION/SENSOR_LAYOUT_AND_CHRACTERIZATION/SET_SENSOR_CALLIBRATION_PARAMETER/SET_CAMERA_SENSOR_PARAM/SET_CAMERA_EXTRINSIC_PARAM ==
  CameraCalibParam : Inport
  INSTALLED_CAMERA_i : ForIterator  IterationLimit=nCameras
  SET_CAMERA_EXTRINSIC_PARAM : Subsystem
  CameraCalibParamSet : Outport
  wires:
  INSTALLED_CAMERA_i/1 -> SET_CAMERA_EXTRINSIC_PARAM/2(SensorID)
  SET_CAMERA_EXTRINSIC_PARAM/1(Out1) -> CameraCalibParamSet/1
  CameraCalibParam/1 -> SET_CAMERA_EXTRINSIC_PARAM/1(SensorParam)

== system Grid_SensorLayout_SpatialAllignment_Clustering/OBJECT_TRACKER_SENSOR_FUSION/SENSOR_LAYOUT_AND_CHRACTERIZATION/SET_SENSOR_CALLIBRATION_PARAMETER/SET_CAMERA_SENSOR_PARAM/SET_CAMERA_INTRINSIC_PARAM ==
  CameraCalibParam : Inport
  CAMERA_TYPE_i : ForIterator  IterationLimit=nCameraTypes
  SET_CAMERA_INTRINSIC_PARAM : Subsystem
  CameraCalibParamSet : Outport
  wires:
  CameraCalibParam/1 -> SET_CAMERA_INTRINSIC_PARAM/1(SensorParam)
  CAMERA_TYPE_i/1 -> SET_CAMERA_INTRINSIC_PARAM/2(SensorID)
  SET_CAMERA_INTRINSIC_PARAM/1(Out1) -> CameraCalibParamSet/1

== system Grid_SensorLayout_SpatialAllignment_Clustering/OBJECT_TRACKER_SENSOR_FUSION/SENSOR_LAYOUT_AND_CHRACTERIZATION/SET_SENSOR_CALLIBRATION_PARAMETER/SET_CAMERA_SENSOR_PARAM/SET_DATA ==
  CameraIntrinsics : Inport
  CameraExtrinsics : Inport  Port=2
  Bus Creator : BusCreator  Inputs=2  OutDataTypeStr=Bus: CAM_SENSOR_PARAM  NonVirtualBus=on
      settings: InheritFromInputs=off
  CAMSnsrParamUpd : Outport
  wires:
  Bus Creator/1 -> CAMSnsrParamUpd/1
  CameraIntrinsics/1 -> Bus Creator/1
  CameraExtrinsics/1 -> Bus Creator/2

== system Grid_SensorLayout_SpatialAllignment_Clustering/OBJECT_TRACKER_SENSOR_FUSION/SENSOR_LAYOUT_AND_CHRACTERIZATION/SET_SENSOR_CALLIBRATION_PARAMETER/SET_RADAR_SENSOR_PARAM/GET_DATA ==
  RADSnsrParam : Inport
  Bus Selector : BusSelector  OutputSignals=RadarIntrinsics,RadarExtrinsics
  <RadarIntrinsics> : Outport
  <RadarExtrinsics> : Outport  Port=2
  wires:
  Bus Selector/1 -> <RadarIntrinsics>/1  "<RadarIntrinsics>"
  RADSnsrParam/1 -> Bus Selector/1
  Bus Selector/2 -> <RadarExtrinsics>/1  "<RadarExtrinsics>"

== system Grid_SensorLayout_SpatialAllignment_Clustering/OBJECT_TRACKER_SENSOR_FUSION/SENSOR_LAYOUT_AND_CHRACTERIZATION/SET_SENSOR_CALLIBRATION_PARAMETER/SET_RADAR_SENSOR_PARAM/SET_DATA ==
  RadarIntrinsics : Inport
  RadarExtrinsics : Inport  Port=2
  Bus Creator : BusCreator  Inputs=2  OutDataTypeStr=Bus: RAD_SENSOR_PARAM  NonVirtualBus=on
      settings: InheritFromInputs=off
  RADSnsrParamUpd : Outport
  wires:
  RadarIntrinsics/1 -> Bus Creator/1  "RadarIntrnsics"
  RadarExtrinsics/1 -> Bus Creator/2  "RadarExtrinsics"
  Bus Creator/1 -> RADSnsrParamUpd/1

== system Grid_SensorLayout_SpatialAllignment_Clustering/OBJECT_TRACKER_SENSOR_FUSION/SENSOR_LAYOUT_AND_CHRACTERIZATION/SET_SENSOR_CALLIBRATION_PARAMETER/SET_RADAR_SENSOR_PARAM/SET_RADAR_EXTRINSIC_PARAM ==
  RadarCalibParam : Inport
  INSTALLED_RADAR_i : ForIterator  IterationLimit=nRadars
  SET_RADAR_EXTRINSIC_PARAM : Subsystem
  RadarCalibParamSet : Outport
  wires:
  RadarCalibParam/1 -> SET_RADAR_EXTRINSIC_PARAM/1(SensorParam)
  INSTALLED_RADAR_i/1 -> SET_RADAR_EXTRINSIC_PARAM/2(SensorID)
  SET_RADAR_EXTRINSIC_PARAM/1(RadarSensorParam) -> RadarCalibParamSet/1

== system Grid_SensorLayout_SpatialAllignment_Clustering/OBJECT_TRACKER_SENSOR_FUSION/SENSOR_LAYOUT_AND_CHRACTERIZATION/SET_SENSOR_CALLIBRATION_PARAMETER/SET_RADAR_SENSOR_PARAM/SET_RADAR_INTRINSIC_PARAM ==
  RadarCalibParam : Inport
  RADAR_TYPE_i : ForIterator  IterationLimit=nRadarTypes
  SET_RADAR_INTRINSIC_PARAM : Subsystem
  RadarCalibParamSet : Outport
  wires:
  RadarCalibParam/1 -> SET_RADAR_INTRINSIC_PARAM/1(SensorParam)
  RADAR_TYPE_i/1 -> SET_RADAR_INTRINSIC_PARAM/2(SensorID)
  SET_RADAR_INTRINSIC_PARAM/1(RadarIntrinsicParam) -> RadarCalibParamSet/1

== system Grid_SensorLayout_SpatialAllignment_Clustering/OBJECT_TRACKER_SENSOR_FUSION/SIMPLIFIED_DBSCAN_FOR_RADAR_MEASUREMENT_GROUPING/DBSCAN_MEASUREMENT_GROUPING/COMPUTE_MEAN_IF_CLUSTER_FORMED/COMPUTE_COVARIANCE ==
  covariance_sum : Inport
  n : Inport  Port=2
  Constant : Constant  Value=uint16(1)
  Constant1 : Constant  Value=uint16(0)
  Constant2 : Constant  Value=single(eye(2))
  Constant3 : Constant  Value=single(0.001)
  Divide : Product  Inputs=*/
  LessThanOrEqual : RelationalOperator  Operator=>  OutDataTypeStr=boolean  RndMeth=Simplest
  LessThanOrEqual1 : RelationalOperator  Operator=<=  OutDataTypeStr=boolean  RndMeth=Simplest
  Logical Operator : Logic  AllPortsSameDT=off  OutDataTypeStr=boolean
  Selector : Selector  NumberOfDimensions=2  InputPortWidth=3  IndexOptions=Index vector (dialog),Index vector (dialog)  Indices=1,1  OutputSizes=1,1
  Selector1 : Selector  NumberOfDimensions=2  InputPortWidth=3  IndexOptions=Index vector (dialog),Index vector (dialog)  Indices=1,1  OutputSizes=1,1
  Subtract : Sum  Inputs=-+
  Switch : Switch  Criteria=u2 > Threshold  Threshold=uint16(1)
  Switch1 : Switch  Criteria=u2 > Threshold  Threshold=uint16(1)
  Covariance : Outport
  wires:
  n/1 -> [nPts], Switch/2
  Constant/1 -> Switch/1
  covariance_sum/1 -> Divide/1
  Constant1/1 -> Switch/3
  Switch/1 -> Subtract/1
  [nPts] -> Subtract/2
  Subtract/1 -> Divide/2
  Logical Operator/1 -> Switch1/2
  Switch1/1 -> Covariance/1
  Constant2/1 -> Switch1/3
  Divide/1 -> Selector1/1, Switch1/1, Selector/1
  Selector/1 -> LessThanOrEqual/1
  Selector1/1 -> LessThanOrEqual1/2
  Constant3/1 -> LessThanOrEqual1/1, LessThanOrEqual/2
  LessThanOrEqual/1 -> Logical Operator/1
  LessThanOrEqual1/1 -> Logical Operator/2

== system Grid_SensorLayout_SpatialAllignment_Clustering/OBJECT_TRACKER_SENSOR_FUSION/SIMPLIFIED_DBSCAN_FOR_RADAR_MEASUREMENT_GROUPING/DBSCAN_MEASUREMENT_GROUPING/COMPUTE_MEAN_IF_CLUSTER_FORMED/COMPUTE_COVARIANCE_SUM ==
  mean : Inport
  MeasArray : Inport  Port=2
  nPoints : Inport  Port=3
  ClusterMembers : Inport  Port=4
  Add1 : Sum
  Bus Selector : BusSelector  OutputSignals=MeasArray
  For Iterator : ForIterator  ResetStates=reset  IterationSource=external
  Matrix Multiply : Product  Multiplication=Matrix(*)
  Selector : Selector  NumberOfDimensions=2  InputPortWidth=3  IndexOptions=Select all,Index vector (port)  Indices=[1 3],1  OutputSizes=1,1
  Selector1 : Selector  NumberOfDimensions=2  InputPortWidth=3  IndexOptions=Select all,Index vector (port)  Indices=[1 3],1  OutputSizes=1,1
  Subtract : Sum  Inputs=+-
  Transpose : Math  Operator=transpose  SaturateOnIntegerOverflow=on
  Unit Delay : UnitDelay  InitialCondition=single(zeros(2,2))  SampleTime=-1
  ClusterCovSUM : Outport
  wires:
  nPoints/1 -> For Iterator/1
  ClusterMembers/1 -> Selector/1
  For Iterator/1 -> Selector/2
  MeasArray/1 -> Bus Selector/1
  Bus Selector/1 -> Selector1/1  "<MeasArray>"
  Selector/1 -> Selector1/2
  Unit Delay/1 -> Add1/1
  Add1/1 -> Unit Delay/1, ClusterCovSUM/1
  Subtract/1 -> Matrix Multiply/1, Transpose/1
  Transpose/1 -> Matrix Multiply/2
  Matrix Multiply/1 -> Add1/2
  Selector1/1 -> Subtract/2
  mean/1 -> Subtract/1

== system Grid_SensorLayout_SpatialAllignment_Clustering/OBJECT_TRACKER_SENSOR_FUSION/SIMPLIFIED_DBSCAN_FOR_RADAR_MEASUREMENT_GROUPING/DBSCAN_MEASUREMENT_GROUPING/COMPUTE_MEAN_IF_CLUSTER_FORMED/COMPUTE_MEAN ==
  mean_sum : Inport
  n : Inport  Port=2
  Divide : Product  Inputs=*/
  mean : Outport
  wires:
  mean_sum/1 -> Divide/1
  Divide/1 -> mean/1
  n/1 -> Divide/2

== system Grid_SensorLayout_SpatialAllignment_Clustering/OBJECT_TRACKER_SENSOR_FUSION/SIMPLIFIED_DBSCAN_FOR_RADAR_MEASUREMENT_GROUPING/DBSCAN_MEASUREMENT_GROUPING/COMPUTE_MEAN_IF_CLUSTER_FORMED/COMPUTE_MEAN_SUM ==
  ClusterMembers : Inport
  nPoints : Inport  Port=2
  MeasArray : Inport  Port=3
  Add1 : Sum
  Bus Selector : BusSelector  OutputSignals=MeasArray
  For Iterator : ForIterator  ResetStates=reset  IterationSource=external
  Selector : Selector  NumberOfDimensions=2  InputPortWidth=3  IndexOptions=Select all,Index vector (port)  Indices=[1 3],1  OutputSizes=1,1
  Selector1 : Selector  NumberOfDimensions=2  InputPortWidth=3  IndexOptions=Select all,Index vector (port)  Indices=[1 3],1  OutputSizes=1,1
  Unit Delay : UnitDelay  InitialCondition=single(0)  SampleTime=-1
  ClusterMeanSUM : Outport
  wires:
  nPoints/1 -> For Iterator/1
  ClusterMembers/1 -> Selector/1
  For Iterator/1 -> Selector/2
  MeasArray/1 -> Bus Selector/1
  Bus Selector/1 -> Selector1/1  "<MeasArray>"
  Selector/1 -> Selector1/2
  Selector1/1 -> Add1/2
  Unit Delay/1 -> Add1/1
  Add1/1 -> ClusterMeanSUM/1, Unit Delay/1

== system Grid_SensorLayout_SpatialAllignment_Clustering/OBJECT_TRACKER_SENSOR_FUSION/SIMPLIFIED_DBSCAN_FOR_RADAR_MEASUREMENT_GROUPING/DBSCAN_MEASUREMENT_GROUPING/COMPUTE_MEAN_IF_CLUSTER_FORMED/GET_DATA ==
  CLSTR : Inport
  Bus Selector : BusSelector  OutputSignals=ClusterSizes,nClusters,ClusterMember
  Selector : Selector  NumberOfDimensions=2  InputPortWidth=3  IndexOptions=Select all,Index vector (port)  Indices=[1 3],1  OutputSizes=1,1
  nPts : Outport
  <ClusterMember> : Outport  Port=2
  wires:
  Bus Selector/1 -> Selector/1  "<ClusterSizes>"
  Selector/1 -> nPts/1
  Bus Selector/2 -> Selector/2  "<nClusters>"
  Bus Selector/3 -> <ClusterMember>/1  "<ClusterMember>"
  CLSTR/1 -> Bus Selector/1

== system Grid_SensorLayout_SpatialAllignment_Clustering/OBJECT_TRACKER_SENSOR_FUSION/SIMPLIFIED_DBSCAN_FOR_RADAR_MEASUREMENT_GROUPING/DBSCAN_MEASUREMENT_GROUPING/FORM_CLUSTER/CHECK_CONDITION ==
  idx_i : Inport
  CLSTR_in : Inport  Port=2
  Bus Selector : BusSelector  OutputSignals=isMeasVisitedFlag
  Logical Operator1 : Logic  Operator=NOT  AllPortsSameDT=off  OutDataTypeStr=boolean
  Selector1 : Selector  NumberOfDimensions=2  InputPortWidth=3  IndexOptions=Select all,Index vector (port)  Indices=1,1  OutputSizes=1,1
  Unit Delay : UnitDelay  InitialCondition=CLSTR_SNSR_DELAY_INIT  SampleTime=-1
  isNotVisited : Outport
  CLSTR_out : Outport  Port=2
  wires:
  Logical Operator1/1 -> isNotVisited/1
  Selector1/1 -> Logical Operator1/1
  idx_i/1 -> Selector1/2
  CLSTR_in/1 -> Unit Delay/1
  Bus Selector/1 -> Selector1/1  "<isMeasVisitedFlag>"
  Unit Delay/1 -> CLSTR_out/1, Bus Selector/1

== system Grid_SensorLayout_SpatialAllignment_Clustering/OBJECT_TRACKER_SENSOR_FUSION/SIMPLIFIED_DBSCAN_FOR_RADAR_MEASUREMENT_GROUPING/DBSCAN_MEASUREMENT_GROUPING/FORM_CLUSTER/DBSCAN ==
  CLSTR_DATA : Inport
  measArray : Inport  Port=2
  idx_i : Inport  Port=3
  Action Port : ActionPort  ActionType=then
  DBSCAN_PROPAGATE_AND_EXPAND_CLUSTER : Subsystem
  INITIALIZE_CLUSTER : Subsystem
  Subsystem : Subsystem
  nPtsEps : Outport
  CLSTR_DATA_UPD : Outport  Port=2
  wires:
  idx_i/1 -> INITIALIZE_CLUSTER/3(idx_i)
  INITIALIZE_CLUSTER/2(CLUSTER_DATA) -> DBSCAN_PROPAGATE_AND_EXPAND_CLUSTER/3(CLSTR_DATA)
  INITIALIZE_CLUSTER/1(nRadMeas) -> DBSCAN_PROPAGATE_AND_EXPAND_CLUSTER/1(nMeas)
  CLSTR_DATA/1 -> INITIALIZE_CLUSTER/1(CLUSTERING_DATA)
  [meas] -> DBSCAN_PROPAGATE_AND_EXPAND_CLUSTER/2(measArray)
  measArray/1 -> INITIALIZE_CLUSTER/2(RAD_MEAS_CTS), [meas]
  DBSCAN_PROPAGATE_AND_EXPAND_CLUSTER/1(CLSTR_DATA_UPD) -> CLSTR_DATA_UPD/1, Subsystem/1(CLSTR_DATA)
  Subsystem/1(ClstrSize) -> nPtsEps/1

== system Grid_SensorLayout_SpatialAllignment_Clustering/OBJECT_TRACKER_SENSOR_FUSION/SIMPLIFIED_DBSCAN_FOR_RADAR_MEASUREMENT_GROUPING/DBSCAN_MEASUREMENT_GROUPING/FORM_CLUSTER/MERGE_SIGNALS ==
  CLSTR_NO_UPD : Inport
  nPtsEpsNoUpd : Inport  Port=2
  nPtsUpd : Inport  Port=3
  CLSTR_UPD : Inport  Port=4
  Merge : Merge
  Merge1 : Merge
  nPtsEps : Outport
  CLSTR_DATA : Outport  Port=2
  wires:
  CLSTR_NO_UPD/1 -> Merge1/1
  Merge1/1 -> CLSTR_DATA/1
  nPtsEpsNoUpd/1 -> Merge/1
  Merge/1 -> nPtsEps/1
  nPtsUpd/1 -> Merge/2
  CLSTR_UPD/1 -> Merge1/2

== system Grid_SensorLayout_SpatialAllignment_Clustering/OBJECT_TRACKER_SENSOR_FUSION/SIMPLIFIED_DBSCAN_FOR_RADAR_MEASUREMENT_GROUPING/DBSCAN_MEASUREMENT_GROUPING/FORM_CLUSTER/NO_CLUSTER_FORMED ==
  CLSTR_DATA : Inport
  Action Port : ActionPort  ActionType=else
  Constant : Constant  Value=uint16(0)
  CLSTR_DATA_NO_UPD : Outport
  nPtsEpsNoUpd : Outport  Port=2
  wires:
  CLSTR_DATA/1 -> CLSTR_DATA_NO_UPD/1
  Constant/1 -> nPtsEpsNoUpd/1

== system Grid_SensorLayout_SpatialAllignment_Clustering/OBJECT_TRACKER_SENSOR_FUSION/SIMPLIFIED_DBSCAN_FOR_RADAR_MEASUREMENT_GROUPING/DBSCAN_MEASUREMENT_GROUPING/MERGE_SIGNALS/GET_DATA_FROM_BUS ==
  CLSTR_DATA : Inport
  Bus Selector : BusSelector  OutputSignals=ClusterCenter,ClusterCovariance,nClusters
  <ClusterCenter> : Outport
  <ClusterCovariance> : Outport  Port=2
  <nClusters> : Outport  Port=3
  wires:
  Bus Selector/3 -> <nClusters>/1  "<nClusters>"
  Bus Selector/1 -> <ClusterCenter>/1  "<ClusterCenter>"
  CLSTR_DATA/1 -> Bus Selector/1
  Bus Selector/2 -> <ClusterCovariance>/1  "<ClusterCovariance>"

== system Grid_SensorLayout_SpatialAllignment_Clustering/OBJECT_TRACKER_SENSOR_FUSION/SIMPLIFIED_DBSCAN_FOR_RADAR_MEASUREMENT_GROUPING/DBSCAN_MEASUREMENT_GROUPING/MERGE_SIGNALS/SET_DATA_TO_BUS ==
  CLSTR_DATA : Inport
  Mean_ARRAY : Inport  Port=2
  Cov_ARRAY : Inport  Port=3
  Bus Creator : BusCreator  Inputs=7  OutDataTypeStr=Bus: CLUSTER_DATA_STRUCT_SNSR  NonVirtualBus=on
      settings: InheritFromInputs=off
  Bus Selector1 : BusSelector  OutputSignals=ClusterCenter,ClusterCovariance,ClusterSizes,ClusterToMeasAssignment,isMeasVisitedFlag,nClusters,ClusterMember
  Constant1 : Constant  Value=ClusterMemArray_SNSR
  Reshape1 : Reshape  OutputDimensionality=Row vector (2-D)
  Terminator1 : Terminator
  Terminator2 : Terminator
  Terminator3 : Terminator
  "CLSTR_DATA_UPD " : Outport
  wires:
  Constant1/1 -> Reshape1/1  "ClusterMember"
  Bus Selector1/5 -> Bus Creator/5  "<isMeasVisitedFlag>"
  Cov_ARRAY/1 -> Bus Creator/2  "ClusterCovariance"
  Mean_ARRAY/1 -> Bus Creator/1  "ClusterCenter"
  Bus Selector1/1 -> Terminator2/1  "<ClusterCenter>"
  Bus Selector1/7 -> Terminator1/1  "<ClusterMember>"
  Bus Selector1/2 -> Terminator3/1  "<ClusterCovariance>"
  Bus Selector1/3 -> Bus Creator/3  "<ClusterSizes>"
  Reshape1/1 -> Bus Creator/7  "ClusterMember"
  Bus Selector1/4 -> Bus Creator/4  "<ClusterToMeasAssignment>"
  Bus Selector1/6 -> Bus Creator/6  "<nClusters>"
  Bus Creator/1 -> "CLSTR_DATA_UPD "/1
  CLSTR_DATA/1 -> Bus Selector1/1

== system Grid_SensorLayout_SpatialAllignment_Clustering/OBJECT_TRACKER_SENSOR_FUSION/SIMPLIFIED_DBSCAN_FOR_RADAR_MEASUREMENT_GROUPING/DBSCAN_MEASUREMENT_GROUPING/MERGE_SIGNALS/UPDATE_CLUSTER_DATA ==
  Center_ARRAY : Inport
  Cov_ARRAY : Inport  Port=2
  ID : Inport  Port=3
  mean1 : Inport  Port=4
  mean2 : Inport  Port=5
  Cov1 : Inport  Port=6
  Cov2 : Inport  Port=7
  FLAG : Inport  Port=8
  Assignment : Assignment  NumberOfDimensions=2  DiagnosticForDimensions=Warning  IndexOptions=Assign all,Index vector (port)  Indices=1,1  OutputSizes=1,1
  Assignment1 : Assignment  NumberOfDimensions=3  DiagnosticForDimensions=Warning  IndexOptions=Assign all,Assign all,Index vector (port)  Indices=1,1,1  OutputSizes=1,1,1
  Merge : Merge
  Merge2 : Merge
  Selector : Selector  NumberOfDimensions=2  InputPortWidth=3  IndexOptions=Select all,Index vector (port)  Indices=[1 3],1  OutputSizes=1,1
  Selector1 : Selector  NumberOfDimensions=3  InputPortWidth=3  IndexOptions=Select all,Select all,Index vector (port)  Indices=[1 3],1,1  OutputSizes=1,1,1
  Switch : Switch  Criteria=u2 ~= 0
  Switch1 : Switch  Criteria=u2 ~= 0
  CenterUpd : Outport
  CovUpd : Outport  Port=2
  wires:
  Selector/1 -> Switch/3
  Merge2/1 -> Switch1/1
  Cov_ARRAY/1 -> Assignment1/1, Selector1/1
  mean1/1 -> Merge/1
  Selector1/1 -> Switch1/3
  Merge/1 -> Switch/1
  Switch1/1 -> Assignment1/2
  Switch/1 -> Assignment/2
  Cov2/1 -> Merge2/2
  Assignment1/1 -> CovUpd/1
  Assignment/1 -> CenterUpd/1
  Cov1/1 -> Merge2/1
  mean2/1 -> Merge/2
  FLAG/1 -> [FLAG]
  [FLAG] -> Switch/2
  [FLAG] -> Switch1/2
  [ID] -> Assignment/3, Selector/2
  ID/1 -> [ID], Assignment1/3, Selector1/2
  Center_ARRAY/1 -> Selector/1, Assignment/1

== system Grid_SensorLayout_SpatialAllignment_Clustering/OBJECT_TRACKER_SENSOR_FUSION/SPATIAL_ALLIGNMENT/CAMERA_MEASUREMENTS_SPATIAL_ALLIGNMENT/For Iterator Subsystem/For Iterator Subsystem ==
  CameraCalibration : Inport
  nMeas : Inport  Port=2
  CameraCAN : Inport  Port=3
  CoordinateTransformation1 : Subsystem  TreatAsAtomicUnit=on
  For Iterator : ForIterator  ResetStates=reset  IterationSource=external
  SetMeasurement1 : Subsystem
  Subsystem : Subsystem
  nValidMeas : Outport
  CameraMeasUpd : Outport  Port=2
  CameraMeasNoiseCovUpd : Outport  Port=3
  CameraMeasRefUpd : Outport  Port=4
  wires:
  nMeas/1 -> For Iterator/1
  CameraCalibration/1 -> CoordinateTransformation1/2(SensorParam)
  CameraCAN/1 -> Subsystem/1(measCAN)
  Subsystem/1(nValidMeasCnt) -> nValidMeas/1
  Subsystem/4(measID) -> SetMeasurement1/3(measID)
  Subsystem/2(isValid) -> CoordinateTransformation1/Action
  CoordinateTransformation1/1(measUpd) -> SetMeasurement1/1(measTransformed)
  For Iterator/1 -> SetMeasurement1/4(CamCANidx), Subsystem/2(measIdx)
  SetMeasurement1/1(CameraCTSMatUpd) -> CameraMeasUpd/1
  SetMeasurement1/2(CameraCTSNoiseCovMatUpd) -> CameraMeasNoiseCovUpd/1
  SetMeasurement1/3(CameraCTSRefUpd) -> CameraMeasRefUpd/1
  Subsystem/3(meas_i) -> CoordinateTransformation1/1(meas), SetMeasurement1/2(CameraMeasCAN)
